simulink model "latFor"  (R2020a)
settings: Solver=VariableStepAuto  StartTime=0.0  StopTime=10  RelTol=1e-3
undefined symbols (not defined in the file or in its folder): A_latFor, B_latFor, C_latFor, IC, K, L
settings Model: Creator=Tomo  LastModifiedBy=Tomo

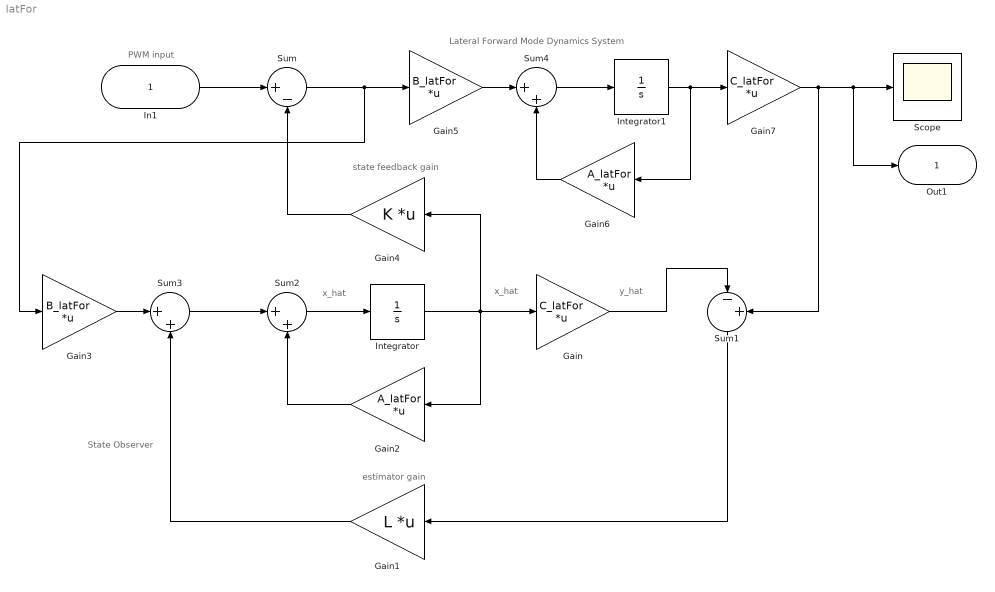
== system latFor ==
  note: State Observer
  note: y_hat
  note: x_hat
  note: x_hat
  note: estimator gain
  note: state feedback gain
  note: Lateral Forward Mode Dynamics System
  note: PWM input
  In1 : Inport
  Gain : Gain  Gain=C_latFor  Multiplication=Matrix(K*u)
  Gain1 : Gain  Gain=L  Multiplication=Matrix(K*u)
  Gain2 : Gain  Gain=A_latFor  Multiplication=Matrix(K*u)
  Gain3 : Gain  Gain=B_latFor  Multiplication=Matrix(K*u)
  Gain4 : Gain  Gain=K  Multiplication=Matrix(K*u)
  Gain5 : Gain  Gain=B_latFor  Multiplication=Matrix(K*u)
  Gain6 : Gain  Gain=A_latFor  Multiplication=Matrix(K*u)
  Gain7 : Gain  Gain=C_latFor  Multiplication=Matrix(K*u)
  Integrator : Integrator  InitialCondition=IC
  Integrator1 : Integrator  InitialCondition=IC
  Scope : Scope
  Sum : Sum  Inputs=|+-
  Sum1 : Sum  Inputs=|-+
  Sum2 : Sum  Inputs=|++
  Sum3 : Sum  Inputs=|++
  Sum4 : Sum  Inputs=|++
  Out1 : Outport
  wires:
  Sum/1 -> Gain5/1, Gain3/1
  Integrator1/1 -> Gain6/1, Gain7/1
  Gain/1 -> Sum1/1
  Sum1/1 -> Gain1/1
  Gain1/1 -> Sum3/2
  Gain2/1 -> Sum2/2
  Sum3/1 -> Sum2/1
  Sum2/1 -> Integrator/1
  Integrator/1 -> Gain2/1, Gain4/1, Gain/1
  Gain4/1 -> Sum/2
  Gain3/1 -> Sum3/1
  Gain5/1 -> Sum4/1
  Sum4/1 -> Integrator1/1
  Gain6/1 -> Sum4/2
  Gain7/1 -> Sum1/2, Out1/1, Scope/1
  In1/1 -> Sum/1
